simulink model "L2_1_sine_sum"  (R2025b)
settings: Solver=VariableStepAuto  StartTime=0.0  StopTime=2  MaxStep=0.01  RelTol=1e-3
settings Model: Creator=kimsteph  LastModifiedBy=kimsteph

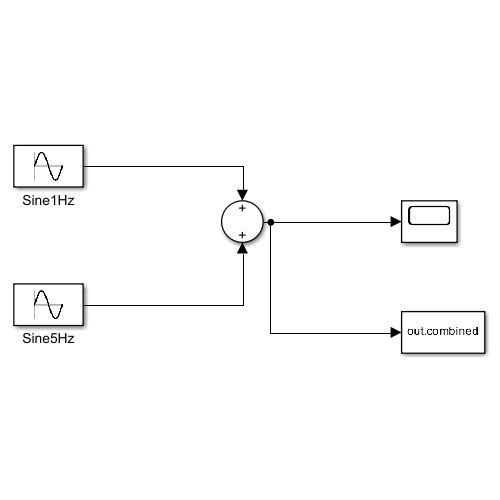
[thumbnail: Simulink's stored preview of the top-level diagram]
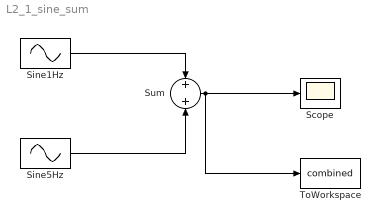
== system L2_1_sine_sum ==
  Scope : Scope
  Sine1Hz : Sin  Frequency=2*pi*1  SampleTime=0
  Sine5Hz : Sin  Amplitude=0.5  Frequency=2*pi*5  SampleTime=0
  Sum : Sum
  ToWorkspace : ToWorkspace  VariableName=combined  SaveFormat=Timeseries  SampleTime=-1
  wires:
  Sine1Hz/1 -> Sum/1
  Sine5Hz/1 -> Sum/2
  Sum/1 -> Scope/1, ToWorkspace/1
